simulink model "joint_space_pd_w_g_comp"  (R2020b)
settings: Solver=FixedStepAuto  StartTime=0.0  StopTime=20  FixedStep=Ts  RelTol=1e-3
values from neighbouring files (symbols this model uses):
  dqi = [0 0 0]'    [main_3DoF_robots.m]
  g_q_c = g_q    [main_3DoF_robots.m]
  he = [fex fey fez uex uey uez]'    [MyRobot.m]    (also in getBHat.m = zeros(6,1); main_3DoF_robots.m = [0 0 0 0 0 0]')
  KD = [10;5;10]    [main_3DoF_robots.m]
  KP = [50;100;50]    [main_3DoF_robots.m]
  myRobot = MyRobot('PRP.urdf', DH, links)    [main_3DoF_robots.m]
  qf = [0.1 pi 0.2]'    [main_3DoF_robots.m]
  qi = [0 0 0]'    [main_3DoF_robots.m]
  Ts = 0.001    [main_3DoF_robots.m]
settings Model: Creator=simon  LastModifiedBy=simon
settings SolverCC: ZeroCrossControl=DisableAll

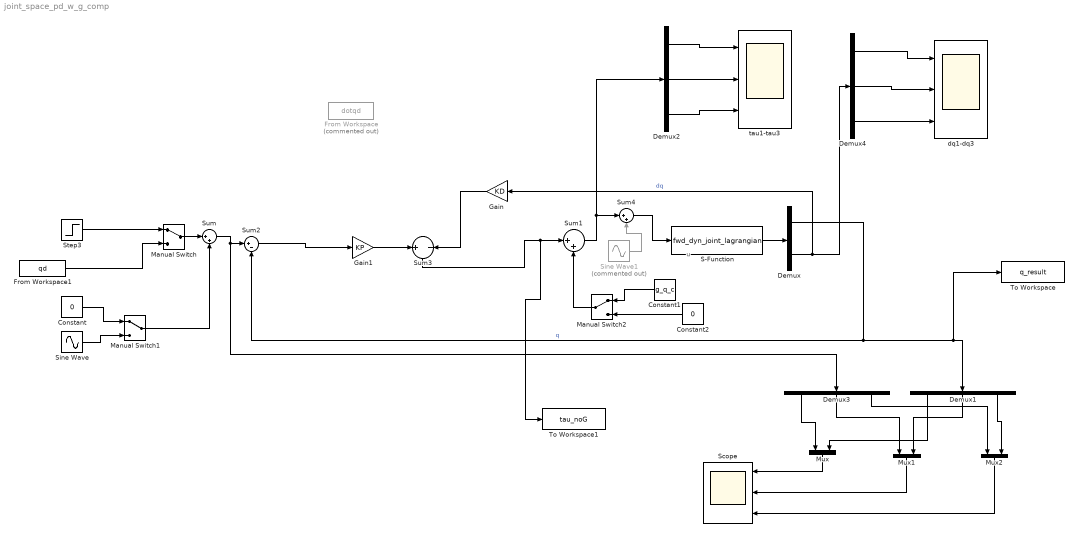
== system joint_space_pd_w_g_comp ==
  note: u
  Constant : Constant  Value=0
  Constant1 : Constant  Value=g_q_c
  Constant2 : Constant  Value=0
  Demux : Demux  Outputs=2
  Demux{1..4} (4 alike) : Demux  Outputs=myRobot.N
  From Workspace : FromWorkspace  Commented=on  VariableName=dotqd  SampleTime=Ts
  From Workspace1 : FromWorkspace  VariableName=qd  SampleTime=Ts
  Gain : Gain  Gain=KD
  Gain1 : Gain  Gain=KP
  Manual Switch : ManualSwitch
  Manual Switch1 : ManualSwitch
  Manual Switch2 : ManualSwitch
  Mux : Mux  Inputs=2
  Mux1 : Mux  Inputs=2
  Mux2 : Mux  Inputs=2
  S-Function : S-Function  FunctionName=fwd_dyn_joint_lagrangian  Parameters=myRobot,he,qi,dqi  SFunctionDeploymentMode=off  EnableBusSupport=off
  Scope : Scope  NumInputPorts=3
  Sine Wave : Sin  Amplitude=0.1  SampleTime=0
  Sine Wave1 : Sin  Commented=on  Amplitude=0.1  Frequency=5  SampleTime=0
  Step3 : Step  Before=qi  After=qf  SampleTime=0
  Sum : Sum  Inputs=|++
  Sum1 : Sum  Inputs=|++
  Sum2 : Sum  Inputs=|+-
  Sum3 : Sum  Inputs=+||-
  Sum4 : Sum  Inputs=|++
  To Workspace : ToWorkspace  VariableName=q_result  SaveFormat=Timeseries  SampleTime=-1
  To Workspace1 : ToWorkspace  VariableName=tau_noG  SaveFormat=Timeseries  SampleTime=-1
  dq1-dq3 : Scope  NumInputPorts=3
  tau1-tau3 : Scope  NumInputPorts=3
  wires:
  Demux2/2 -> tau1-tau3/2
  Demux/1 -> Sum2/2, To Workspace/1, Demux1/1  "q"
  Sum3/1 -> To Workspace1/1, Sum1/1
  Demux2/1 -> tau1-tau3/1
  S-Function/1 -> Demux/1
  Demux2/3 -> tau1-tau3/3
  Sum1/1 -> Sum4/1, Demux2/1
  Demux/2 -> Demux4/1, Gain/1  "dq"
  Sum2/1 -> Gain1/1
  Gain1/1 -> Sum3/1
  Gain/1 -> Sum3/2
  Demux4/3 -> dq1-dq3/3
  Demux4/2 -> dq1-dq3/2
  Demux4/1 -> dq1-dq3/1
  Manual Switch/1 -> Sum/1
  Demux3/1 -> Mux/1
  Demux1/1 -> Mux/2
  Demux3/2 -> Mux1/1
  Demux1/2 -> Mux1/2
  Demux3/3 -> Mux2/1
  Demux1/3 -> Mux2/2
  Mux/1 -> Scope/1
  Mux1/1 -> Scope/2
  Mux2/1 -> Scope/3
  Step3/1 -> Manual Switch/1
  From Workspace1/1 -> Manual Switch/2
  Constant/1 -> Manual Switch1/1
  Sine Wave/1 -> Manual Switch1/2
  Sum/1 -> Demux3/1, Sum2/1
  Manual Switch1/1 -> Sum/2
  Manual Switch2/1 -> Sum1/2
  Constant1/1 -> Manual Switch2/1
  Constant2/1 -> Manual Switch2/2
  Sum4/1 -> S-Function/1
  Sine Wave1/1 -> Sum4/2
